simulink model "impedance_control"  (R2020b)
settings: Solver=VariableStepAuto  StartTime=0.0  StopTime=2.0  RelTol=1e-3
undefined symbols (not defined in the file or in its folder): qn, qn_dot
settings Model: Creator=Jae  LastModifiedBy=Jae

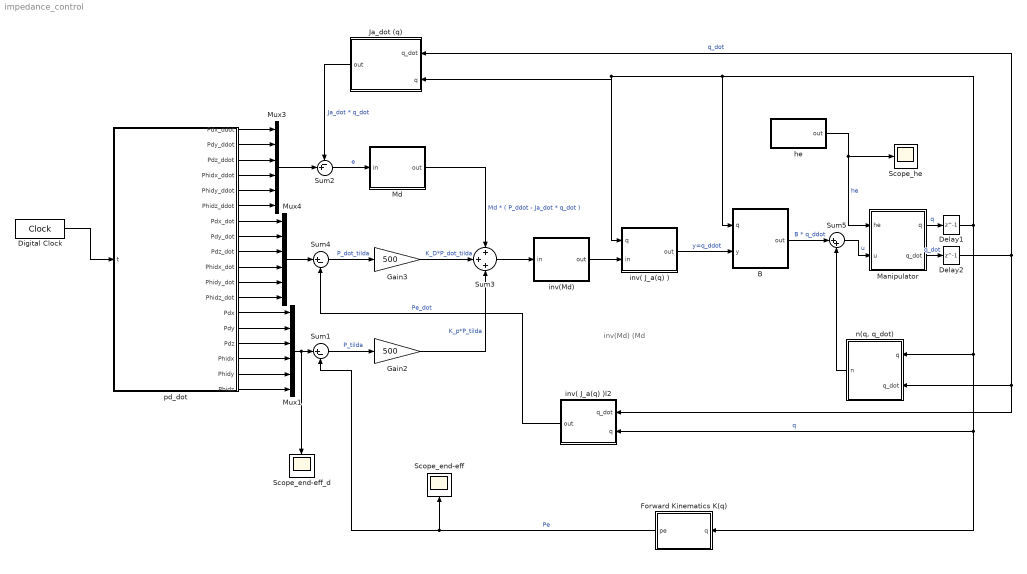
== system impedance_control ==
  note: inv(Md) (Md
  B : MATLAB Function  TreatAsAtomicUnit=on
  Delay1 : Delay  DelayLength=1  InitialCondition=[1 2 3 qn]';
  Delay2 : Delay  DelayLength=1  InitialCondition=[1 2 3 qn_dot]';
  Digital Clock : DigitalClock  SampleTime=0.01
  Forward Kinematics K(q) : MATLAB Function  TreatAsAtomicUnit=on
  Gain2 : Gain  Gain=500
  Gain3 : Gain  Gain=500
  Ja_dot (q) : MATLAB Function  TreatAsAtomicUnit=on
  Manipulator : Subsystem
  Md : MATLAB Function  TreatAsAtomicUnit=on
  Mux1 : Mux  Inputs=6
  Mux3 : Mux  Inputs=6
  Mux4 : Mux  Inputs=6
  Scope_end-eff : Scope
  Scope_end-eff_d : Scope
  Scope_he : Scope
  Sum1 : Sum  Inputs=|+-
  Sum2 : Sum  Inputs=-+|
  Sum3 : Sum  Inputs=+++
  Sum4 : Sum  Inputs=|+-
  Sum5 : Sum  Inputs=|++
  he : MATLAB Function  TreatAsAtomicUnit=on
  inv( J_a(q) ) : MATLAB Function  TreatAsAtomicUnit=on
  inv( J_a(q) )l2 : MATLAB Function  TreatAsAtomicUnit=on
  inv(Md) : MATLAB Function  TreatAsAtomicUnit=on
  "n(q, q_dot)" : Subsystem
  pd_dot : MATLAB Function  TreatAsAtomicUnit=on
  wires:
  Digital Clock/1 -> pd_dot/1(t)
  inv( J_a(q) )/1(out) -> B/2(y)  "y=q_ddot"
  pd_dot/13(Pdx) -> Mux1/1
  pd_dot/14(Pdy) -> Mux1/2
  pd_dot/15(Pdz) -> Mux1/3
  pd_dot/16(Phidx) -> Mux1/4
  pd_dot/17(Phidy) -> Mux1/5
  pd_dot/18(Phidz) -> Mux1/6
  pd_dot/1(Pdx_ddot) -> Mux3/1
  pd_dot/2(Pdy_ddot) -> Mux3/2
  pd_dot/3(Pdz_ddot) -> Mux3/3
  pd_dot/4(Phidx_ddot) -> Mux3/4
  pd_dot/5(Phidy_ddot) -> Mux3/5
  pd_dot/6(Phidz_ddot) -> Mux3/6
  pd_dot/7(Pdx_dot) -> Mux4/1
  pd_dot/8(Pdy_dot) -> Mux4/2
  pd_dot/9(Pdz_dot) -> Mux4/3
  pd_dot/10(Phidx_dot) -> Mux4/4
  pd_dot/11(Phidy_dot) -> Mux4/5
  pd_dot/12(Phidz_dot) -> Mux4/6
  Gain3/1 -> Sum3/2  "K_D*P_dot_tilda"
  Mux3/1 -> Sum2/2
  Sum2/1 -> Md/1(in)  "e"
  Md/1(out) -> Sum3/1  "Md * ( P_ddot - Ja_dot * q_dot )"
  Mux4/1 -> Sum4/1
  Sum4/1 -> Gain3/1  "P_dot_tilda"
  Mux1/1 -> Scope_end-eff_d/1, Sum1/1
  Sum1/1 -> Gain2/1  "P_tilda"
  Sum3/1 -> inv(Md)/1(in)
  Gain2/1 -> Sum3/3  "K_p*P_tilda"
  inv(Md)/1(out) -> inv( J_a(q) )/2(in)
  Ja_dot (q)/1(out) -> Sum2/1  "Ja_dot * q_dot"
  Forward Kinematics K(q)/1(pe) -> Scope_end-eff/1, Sum1/2  "Pe"
  inv( J_a(q) )l2/1(out) -> Sum4/2  "Pe_dot"
  B/1(out) -> Sum5/1  "B * q_ddot"
  "n(q, q_dot)"/1(n) -> Sum5/2
  Manipulator/1(q) -> Delay1/1  "q"
  Delay1/1 -> "n(q, q_dot)"/1(q), inv( J_a(q) )l2/2(q), Forward Kinematics K(q)/1(q), B/1(q), inv( J_a(q) )/1(q), Ja_dot (q)/2(q)  "q"
  Manipulator/2(q_dot) -> Delay2/1  "q_dot"
  Delay2/1 -> inv( J_a(q) )l2/1(q_dot), "n(q, q_dot)"/2(q_dot), Ja_dot (q)/1(q_dot)  "q_dot"
  Sum5/1 -> Manipulator/2(u)  "u"
  he/1(out) -> Scope_he/1, Manipulator/1(he)  "he"

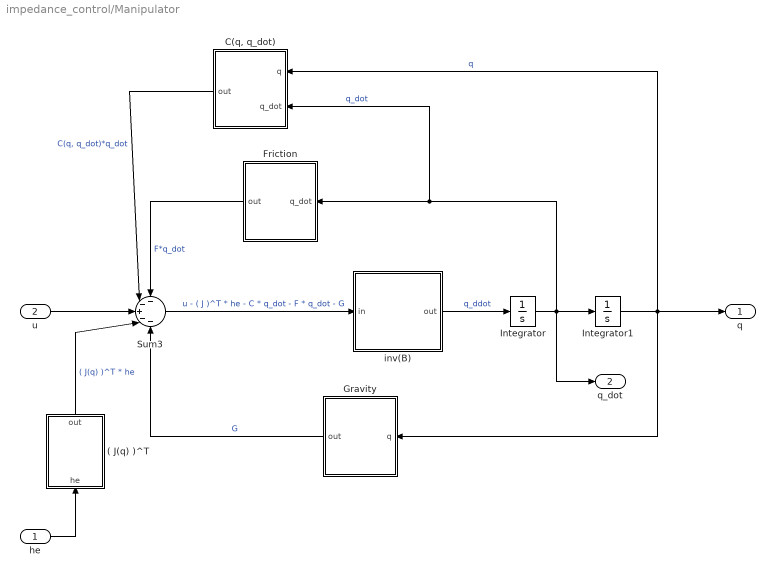
== system impedance_control/Manipulator ==
  he : Inport
  u : Inport  Port=2
  ( J(q) )^T : MATLAB Function  TreatAsAtomicUnit=on
  "C(q, q_dot)" : MATLAB Function  TreatAsAtomicUnit=on
  Friction : MATLAB Function  TreatAsAtomicUnit=on
  Gravity : MATLAB Function  TreatAsAtomicUnit=on
  Integrator : Integrator  InitialCondition=[0 0]  ZeroCross=off
  Integrator1 : Integrator  InitialCondition=[0 0]  ZeroCross=off
  Sum3 : Sum  Inputs=--+--
  inv(B) : MATLAB Function  TreatAsAtomicUnit=on
  q : Outport
  q_dot : Outport  Port=2
  wires:
  u/1 -> Sum3/3
  ( J(q) )^T/1(out) -> Sum3/4  "( J(q) )^T * he"
  "C(q, q_dot)"/1(out) -> Sum3/2  "C(q, q_dot)*q_dot"
  Friction/1(out) -> Sum3/1  "F*q_dot"
  inv(B)/1(out) -> Integrator/1  "q_ddot"
  Integrator/1 -> Integrator1/1, q_dot/1, Friction/1(q_dot), "C(q, q_dot)"/2(q_dot)  "q_dot"
  Integrator1/1 -> Gravity/1(q), "C(q, q_dot)"/1(q), q/1  "q"
  Sum3/1 -> inv(B)/1(in)  "u - ( J )^T * he - C * q_dot - F * q_dot - G"
  Gravity/1(out) -> Sum3/5  "G"
  he/1 -> ( J(q) )^T/1(he)

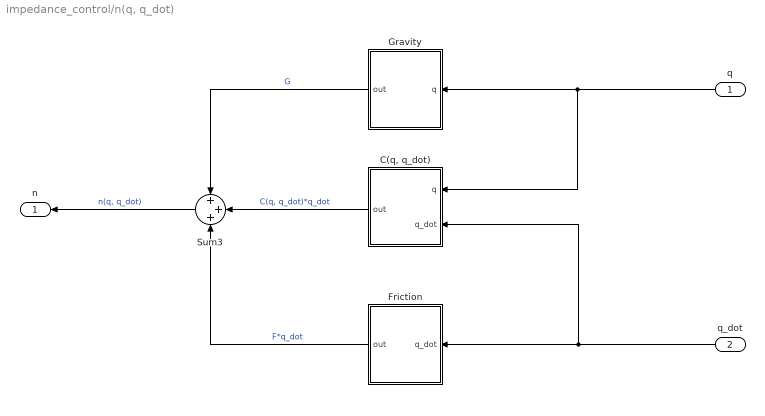
== system impedance_control/n(q, q_dot) ==
  q : Inport
  q_dot : Inport  Port=2
  "C(q, q_dot)" : MATLAB Function  TreatAsAtomicUnit=on
  Friction : MATLAB Function  TreatAsAtomicUnit=on
  Gravity : MATLAB Function  TreatAsAtomicUnit=on
  Sum3 : Sum  Inputs=+++
  n : Outport
  wires:
  Sum3/1 -> n/1  "n(q, q_dot)"
  Gravity/1(out) -> Sum3/1  "G"
  "C(q, q_dot)"/1(out) -> Sum3/2  "C(q, q_dot)*q_dot"
  Friction/1(out) -> Sum3/3  "F*q_dot"
  q/1 -> "C(q, q_dot)"/1(q), Gravity/1(q)
  q_dot/1 -> "C(q, q_dot)"/2(q_dot), Friction/1(q_dot)

== matlab function impedance_control/inv( J_a(q) )l2 ==
  data: q_dot input; out output; q input
function out = Ja(q_dot, q)
% need to calculate Ja using q
Ja = [];

out = Ja*q_dot;
end

== matlab function impedance_control/n(q, q_dot)/C(q, q_dot) ==
  data: q input; q_dot input; out output
function out = C(q,q_dot)
% need to calculate C
C=[];
out=C*q_dot;
end

== matlab function impedance_control/n(q, q_dot)/Gravity ==
  data: q input; out output
function out = G(q)
% G Calculation
G=[];
out=G;
end

== matlab function impedance_control/n(q, q_dot)/Friction ==
  data: q_dot input; out output
function out = F(q_dot)
% need to define F
F=[1];
out=F*q_dot;
end

== matlab function impedance_control/he ==
  data: out output
function out = he()
% need to define user input he
he=[];
out=he;
end

== matlab function impedance_control/Manipulator/( J(q) )^T ==
  data: out output; he input
function out = J_T(he)
% need to define he 6x1 he

% need to calculate J 6xn
J=[];
    % nx6 * 6x1 
out = J'*he;
end

== matlab function impedance_control/Manipulator/C(q, q_dot) ==
  data: q input; q_dot input; out output
function out = C(q,q_dot)
% need to calculate C
C=[];
out=C*q_dot;
end

== matlab function impedance_control/Manipulator/Friction ==
  data: q_dot input; out output
function out = F(q_dot)
% need to define F
F=[1];
out=F*q_dot;
end

== matlab function impedance_control/Manipulator/Gravity ==
  data: q input; out output
function out = G(q)
% G Calculation
G=[];
out=G;
end

== matlab function impedance_control/B ==
  data: q input; y input; out output
function out = B(q, y)
% need to calculate B using q

B=[];
out=B*y;
end

== matlab function impedance_control/Md ==
  data: in input; out output
% Multiply by Md
function out = Md(in)
% 6x6 matrix
% user input
input=[2 1 1 2 5 7];
Md = diag(input);
                        %6x6 * (6x1+6x1)
out = Md * in;
end

== matlab function impedance_control/inv(Md) ==
  data: in input; out output
% Multiply by inv(Md)
function out = invMd(in)
% user input
input=[2 1 1 2 5 7];

Md = diag(input);
% psuedo-inverse just in case when Md is not 6x6 mat
out = pinv(Md)*in;
end

== matlab function impedance_control/Ja_dot (q) ==
  data: q_dot input; out output; q input
function out = Ja_dot(q_dot, q)
% need to calculate Ja_dot using q
Ja_dot = [];

out = Ja_dot*q_dot;
end

== matlab function impedance_control/pd_dot ==
  data: Pdx_ddot output; Pdy_ddot output; Pdz_ddot output; Phidx_ddot output; Phidy_ddot output; Phidz_ddot output; Pdx_dot output; Pdy_dot output; Pdz_dot output; Phidx_dot output; Phidy_dot output; Phidz_dot output; t input; Pdx output; Pdy output; Pdz output; Phidx output; Phidy output; Phidz output
function [Pdx_ddot,Pdy_ddot,Pdz_ddot,Phidx_ddot,Phidy_ddot,Phidz_ddot,Pdx_dot,Pdy_dot,Pdz_dot,Phidx_dot,Phidy_dot,Phidz_dot,Pdx,Pdy,Pdz,Phidx,Phidy,Phidz] = pos_vel_acc(t)
% Pd
Pdx=sin(t);
Pdy=cos(t);
Pdz=0;
Phidx=0;
Phidy=0;
Phidz=0;
% Pd_dot
Pdx_dot=diff(Pdx,t);
Pdy_dot=diff(Pdy,t);
Pdz_dot=diff(Pdz,t);
Phidx_dot=diff(Phidx,t);
Phidy_dot=diff(Phidy,t);
Phidz_dot=diff(Phidz,t);
% Pd_ddot
Pdx_ddot=diff(Pdx_dot,t);
Pdy_ddot=diff(Pdy_dot,t);
Pdz_ddot=diff(Pdz_dot,t);
Phidx_ddot=diff(Phidx_dot,t);
Phidy_ddot=diff(Phidy_dot,t);
Phidz_ddot=diff(Phidz_dot,t);
end

== matlab function impedance_control/Manipulator/inv(B) ==
  data: in input; out output
function out = invB(in)
% need to calculate B
B=[];
out=pinv(B)*in;
end

== matlab function impedance_control/Forward Kinematics K(q) ==
  data: q input; pe output
function pe = f_kin(q)
if isempty(q)==1
    q = [-2.8210 -2.9561 6.5625];
end
pe = ;
end

== matlab function impedance_control/inv( J_a(q) ) ==
  data: q input; in input; out output
function out = invJa(q, in)
% need to calculate Ja using q
Ja = [];

out = pinv(Ja)*in;
end
